simulink model "BB2"  (Simulink 7.3)
settings: Solver=FixedStepDiscrete  SolverMode=SingleTasking  StartTime=0.0  StopTime=870  RelTol=1e-3
PreLoadFcn:
  | if ~exist('Bund')
  | [data,txt]=xlsread('BundDaily.xls');
  | Bund=data(:,end);
  | end
libraries: dspbuff3 x3, dspstat3 x2, dspsrcs4 x1
settings Model: Creator=kassama  LastModifiedBy=kassama
settings DataIOCC: SaveOutput=off  SignalLogging=off  SaveTime=off
settings OptimizationCC: InitFltsAndDblsToZero=on
settings DebuggingCC: AlgebraicLoopMsg=error  SingleTaskRateTransMsg=error

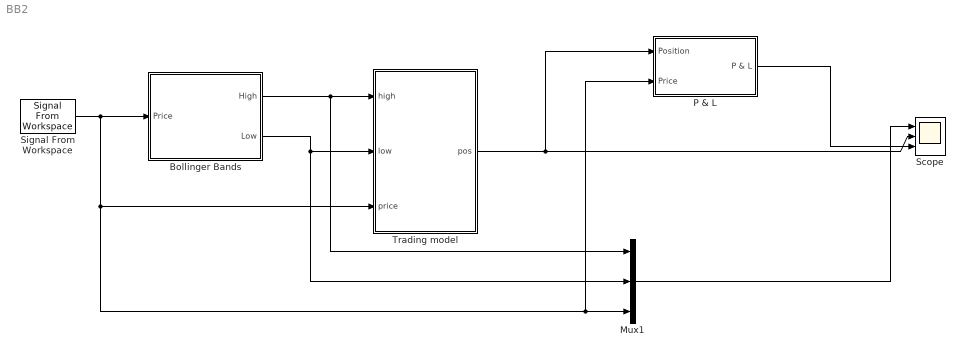
== system BB2 ==
  Bollinger Bands : Subsystem  mask{wlen=50}
      mask prompts: wlen "window length"
  Mux1 : Mux  Inputs=3
  P & L : Subsystem
  Scope : Scope  NumInputPorts=3
      settings: YMin=113.5~-1~0.1  YMax=122~1~1.4
  Signal From Workspace : dspsrcs4/Signal From Workspace  SystemSampleTime=-1  X=Bund  Ts=1  nsamps=1  OutputAfterFinalValue=Setting to zero  ignoreOrWarnInputAndFrameLengths=off
  Trading model : Stateflow chart
  wires:
  Signal From Workspace/1 -> Bollinger Bands/1(Price), Trading model/3(price), Mux1/3, P & L/2(Price)
  Bollinger Bands/1(High) -> Trading model/1(high), Mux1/1
  Bollinger Bands/2(Low) -> Trading model/2(low), Mux1/2
  Trading model/1(pos) -> P & L/1(Position), Scope/2
  P & L/1(P & L) -> Scope/3
  Mux1/1 -> Scope/1

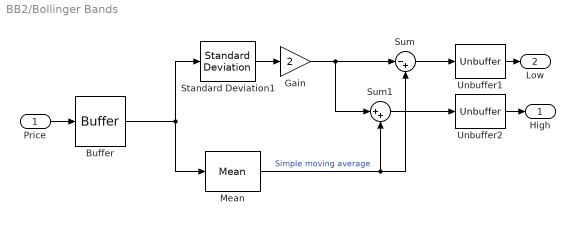
== system BB2/Bollinger Bands ==
  Price : Inport  OutDataType=sfix(16)  OutScaling=2^0
  Buffer : dspbuff3/Buffer  N=wlen  V=wlen-1  ic=0
  Gain : Gain  Gain=2  ParameterDataType=sfix(16)  ParameterScaling=2^0  OutDataType=sfix(16)  OutScaling=2^0
  Mean : dspstat3/Mean  DialogController=dspDDGCreate  DialogControllerArgs=DataTag0  run=off  reset_popup=None  directionMode=Each column  dimension=1  treatSBRowAsCol=on  roiEnable=off  roiType=Rectangles  roiPortion=Entire ROI  roiOutput=Individual statistics for each ROI  roiFlag=off  roundingMode=Floor  overflowMode=off
  Standard Deviation1 : dspstat3/Standard Deviation  DialogController=dspDDGCreate  DialogControllerArgs=DataTag1  run=off  reset_popup=None  directionMode=Each column  dimension=1  treatSBRowAsCol=on  roiEnable=off  roiType=Rectangles  roiPortion=Entire ROI  roiOutput=Individual statistics for each ROI  roiFlag=off
  Sum : Sum  Inputs=|-+  OutDataType=sfix(16)  OutScaling=2^0
  Sum1 : Sum  Inputs=|++  OutDataType=sfix(16)  OutScaling=2^0
  Unbuffer1 : dspbuff3/Unbuffer  ic=0
  Unbuffer2 : dspbuff3/Unbuffer  ic=0
  High : Outport  OutDataType=sfix(16)  OutScaling=2^0
  Low : Outport  Port=2  OutDataType=sfix(16)  OutScaling=2^0
  wires:
  Unbuffer1/1 -> Low/1
  Unbuffer2/1 -> High/1
  Gain/1 -> Sum1/1, Sum/1
  Sum1/1 -> Unbuffer2/1
  Sum/1 -> Unbuffer1/1
  Standard Deviation1/1 -> Gain/1
  Mean/1 -> Sum1/2, Sum/2  "Simple moving average"
  Buffer/1 -> Standard Deviation1/1, Mean/1
  Price/1 -> Buffer/1

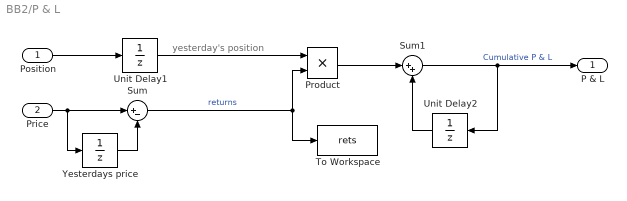
== system BB2/P & L ==
  note: yesterday's position
  Position : Inport  OutDataType=sfix(16)  OutScaling=2^0
  Price : Inport  Port=2  OutDataType=sfix(16)  OutScaling=2^0
  Product : Product  OutDataType=sfix(16)  OutScaling=2^0  RndMeth=Zero
  Sum : Sum  Inputs=|+-  OutDataType=sfix(16)  OutScaling=2^0
  Sum1 : Sum  Inputs=|++  OutDataType=sfix(16)  OutScaling=2^0
  To Workspace : ToWorkspace  VariableName=rets  SampleTime=-1  SaveFormat=Array
  Unit Delay1 : UnitDelay  SampleTime=-1
  Unit Delay2 : UnitDelay  SampleTime=-1
  Yesterdays price : UnitDelay  X0=Bund(2)  SampleTime=-1
  P & L : Outport  OutDataType=sfix(16)  OutScaling=2^0
  wires:
  Sum1/1 -> Unit Delay2/1, P & L/1  "Cumulative P & L"
  Unit Delay2/1 -> Sum1/2
  Yesterdays price/1 -> Sum/2
  Product/1 -> Sum1/1
  Unit Delay1/1 -> Product/1
  Sum/1 -> To Workspace/1, Product/2  "returns"
  Price/1 -> Yesterdays price/1, Sum/1
  Position/1 -> Unit Delay1/1

== stateflow chart Trading model ==
  state Flat
    en:pos=0;
  state long
    en:pos=1;
  state short
    en:pos=-1;
  state Burn_In
    en:count=0;
    du:count+=1;
  (junction 7) -> short [order 1] : [price>high]
  Flat -> (junction 7) : {mid=0.5*(low+high);}
  (junction 7) -> long [order 2] : [price<low]
  (default) -> Burn_In
  long -> Flat : [price>=0.5*(mid+low)]
  short -> Flat : [price<=0.5*(mid+high)]
  (junction 7) -> Flat [order 3]
  Burn_In -> Flat : [count>49]
  data: count local double size=1; high input double; low input double; price input double; pos output double; mid local double
